simulink model "esercizio1sim"  (R2018a)
settings: Solver=ode45  StartTime=0.0  StopTime=10.0  RelTol=1e-3  EnableMultiTasking=on
values from neighbouring files (symbols this model uses):
  A = [2 1 -1; -3 -2 -1; -1 1 -4]    [esercizio1mat.m]    (also in esercizio2mat.m = [0 1 0 0; esercizio3mat.m = [1 1 0; -5 -3 0; 2 3 -1])
  b = [1 0 1]'    [esercizio1mat.m]    (also in esercizio3mat.m = [1; 1; 0])
  c = [0 0 1]    [esercizio1mat.m]    (also in esercizio3mat.m = [1 1 1])
  K = 1/guadagnochiuso; disp(guadagnochiuso)    [esercizio1mat.m]
  k = acker(A, -b, autovalori); disp(k)    [esercizio1mat.m]    (also in esercizio2mat.m = acker(A, -B, autov_controllore); disp(k))
  l = lT'; disp(l)    [esercizio1mat.m]    (also in esercizio2mat.m)
libraries: simulink x2
settings Model: Creator=Fabio  LastModifiedBy=Matteo
settings DataIOCC: LimitDataPoints=on  SaveFormat=Array  SignalLoggingSaveFormat=ModelDataLogs
settings OptimizationCC: ExpressionDepthLimit=2147483647  LifeSpan=inf
settings DebuggingCC: UnderspecifiedInitializationDetection=Classic  MergeDetectMultiDrivingBlocksExec=none  SolverPrmCheckMsg=warning  FcnCallInpInsideContextMsg=warning  StateNameClashWarn=warning  SFUnexpectedBacktrackingDiag=warning  SFNoUnconditionalDefaultTransitionDiag=warning  SFExecutionAtInitializationDiag=none
settings HardwareCC: ProdBitPerPointer=32  ProdBitPerSizeT=32  ProdBitPerPtrDiffT=32  ProdLargestAtomicFloat=None  ProdIntDivRoundTo=Undefined  ProdEndianess=Unspecified  ProdWordSize=32  ProdHWDeviceType=32-bit Generic
settings ModelReferenceCC: PropagateSignalLabelsOutOfModel=off
settings CodeAppCC: StateflowObjectComments=on
settings GRTTargetCC: TargetLangStandard=C89/C90 (ANSI)  GeneratePreprocessorConditionals=Disable all  CombineOutputUpdateFcns=off  GRTInterface=on
settings ConfigComp: CovMetricSettings=dw  CovHtmlReporting=on  CovSaveCumulativeToWorkspaceVar=on  CovSaveSingleToWorkspaceVar=on  CovExternalEMLEnable=off

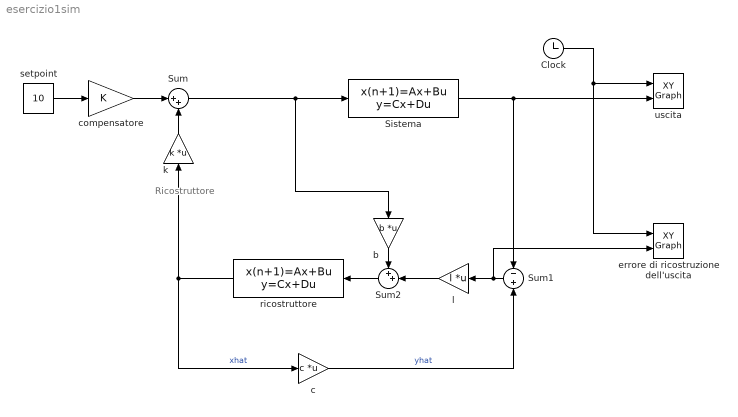
== system esercizio1sim ==
  note: Ricostruttore
  Clock : Clock
  Sistema : DiscreteStateSpace  A=A  B=b  C=c  D=0  InitialCondition=randn(3,1)
  Sum : Sum  Inputs=|++
  Sum1 : Sum  Inputs=-|+
  Sum2 : Sum  Inputs=++|
  b : Gain  Gain=b  Multiplication=Matrix(K*u)
  c : Gain  Gain=c  Multiplication=Matrix(K*u)
  compensatore : Gain  Gain=K
  errore di ricostruzione dell'uscita : simulink/Sinks/XY Graph  xmin=0  xmax=10  ymin=-20  ymax=20  st=-1
  k : Gain  Gain=k  Multiplication=Matrix(K*u)
  l : Gain  Gain=l  Multiplication=Matrix(K*u)
  ricostruttore : DiscreteStateSpace  A=A  B=eye(3)  C=eye(3)  D=zeros(3)  InitialCondition=randn(3,1)
  setpoint : Constant  Value=10  VectorParams1D=off
  uscita : simulink/Sinks/XY Graph  xmin=0  xmax=10  ymin=-20  ymax=20  st=-1
  wires:
  Sistema/1 -> Sum1/1, uscita/2
  Clock/1 -> errore di ricostruzione dell'uscita/1, uscita/1
  setpoint/1 -> compensatore/1
  ricostruttore/1 -> c/1, k/1  "xhat"
  c/1 -> Sum1/2  "yhat"
  Sum1/1 -> errore di ricostruzione dell'uscita/2, l/1
  b/1 -> Sum2/1
  l/1 -> Sum2/2
  Sum2/1 -> ricostruttore/1
  k/1 -> Sum/2
  compensatore/1 -> Sum/1
  Sum/1 -> b/1, Sistema/1
